simulink model "One_Stage"  (R2019b)
settings: Solver=VariableStepAuto  StartTime=0.0  StopTime=10.0  RelTol=1e-3
undefined symbols (not defined in the file): alpha, beta, hyperparameters, sigmaF, sigmaL, XFit
settings Model: Creator=licem  LastModifiedBy=licem

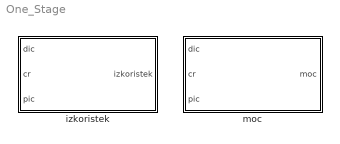
== system One_Stage ==
  izkoristek : Subsystem
  moc : Subsystem

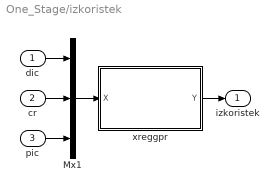
== system One_Stage/izkoristek ==
  dic : Inport
  cr : Inport  Port=2
  pic : Inport  Port=3
  Mx1 : Mux  Inputs=3
  xreggpr : Subsystem
      mask init:
      | xregmaskinitialization;
  izkoristek : Outport
  wires:
  dic/1 -> Mx1/1
  cr/1 -> Mx1/2
  pic/1 -> Mx1/3
  Mx1/1 -> xreggpr/1(X)
  xreggpr/1(Y) -> izkoristek/1

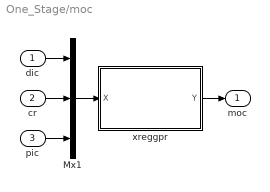
== system One_Stage/moc ==
  dic : Inport
  cr : Inport  Port=2
  pic : Inport  Port=3
  Mx1 : Mux  Inputs=3
  xreggpr : Subsystem
      mask init:
      | xregmaskinitialization;
  moc : Outport
  wires:
  dic/1 -> Mx1/1
  cr/1 -> Mx1/2
  pic/1 -> Mx1/3
  Mx1/1 -> xreggpr/1(X)
  xreggpr/1(Y) -> moc/1

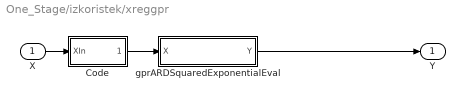
== system One_Stage/izkoristek/xreggpr ==
  X : Inport
  Code : Subsystem
  gprARDSquaredExponentialEval : Subsystem
  Y : Outport
  wires:
  X/1 -> Code/1(XIn)
  Code/1(XCoded) -> gprARDSquaredExponentialEval/1(X)
  gprARDSquaredExponentialEval/1(Y) -> Y/1

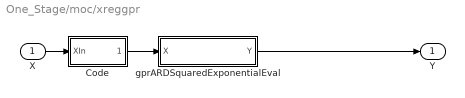
== system One_Stage/moc/xreggpr ==
  X : Inport
  Code : Subsystem
  gprARDSquaredExponentialEval : Subsystem
  Y : Outport
  wires:
  X/1 -> Code/1(XIn)
  Code/1(XCoded) -> gprARDSquaredExponentialEval/1(X)
  gprARDSquaredExponentialEval/1(Y) -> Y/1

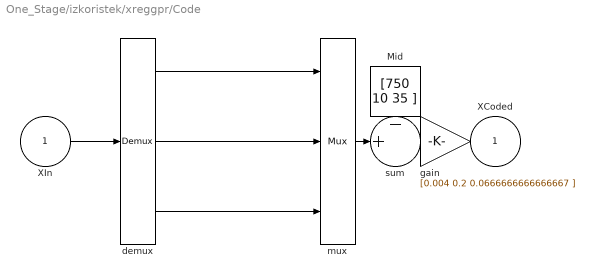
== system One_Stage/izkoristek/xreggpr/Code ==
  XIn : Inport
  Mid : Constant  Value=[750 10 35 ]
  demux : Demux  Outputs=3
  gain : Gain  Gain=[0.004 0.2 0.0666666666666667 ]  SaturateOnIntegerOverflow=on  OutDataTypeStr=Inherit: Same as input  ParamDataTypeStr=Inherit: Same as input
  mux : Mux  Inputs=3
  sum : Sum  Inputs=-+|  SaturateOnIntegerOverflow=on  InputSameDT=on  OutDataTypeStr=Inherit: Same as first input
  XCoded : Outport
  wires:
  demux/1 -> mux/1
  demux/2 -> mux/2
  demux/3 -> mux/3
  Mid/1 -> sum/1
  XIn/1 -> demux/1
  mux/1 -> sum/2
  sum/1 -> gain/1
  gain/1 -> XCoded/1

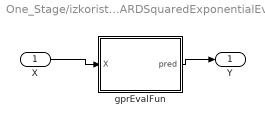
== system One_Stage/izkoristek/xreggpr/gprARDSquaredExponentialEval ==
  X : Inport
  gprEvalFun : MATLAB Function  TreatAsAtomicUnit=on
  Y : Outport
  wires:
  X/1 -> gprEvalFun/1(X)
  gprEvalFun/1(pred) -> Y/1

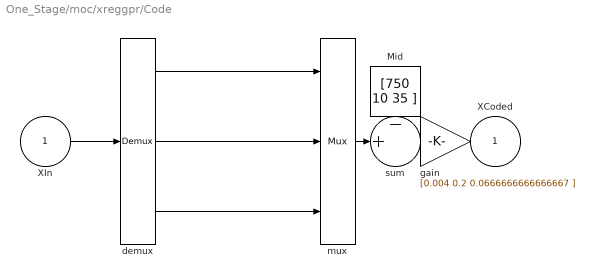
== system One_Stage/moc/xreggpr/Code ==
  XIn : Inport
  Mid : Constant  Value=[750 10 35 ]
  demux : Demux  Outputs=3
  gain : Gain  Gain=[0.004 0.2 0.0666666666666667 ]  SaturateOnIntegerOverflow=on  OutDataTypeStr=Inherit: Same as input  ParamDataTypeStr=Inherit: Same as input
  mux : Mux  Inputs=3
  sum : Sum  Inputs=-+|  SaturateOnIntegerOverflow=on  InputSameDT=on  OutDataTypeStr=Inherit: Same as first input
  XCoded : Outport
  wires:
  demux/1 -> mux/1
  demux/2 -> mux/2
  demux/3 -> mux/3
  Mid/1 -> sum/1
  XIn/1 -> demux/1
  mux/1 -> sum/2
  sum/1 -> gain/1
  gain/1 -> XCoded/1

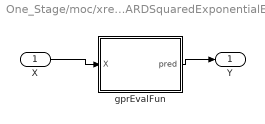
== system One_Stage/moc/xreggpr/gprARDSquaredExponentialEval ==
  X : Inport
  gprEvalFun : MATLAB Function  TreatAsAtomicUnit=on
  Y : Outport
  wires:
  X/1 -> gprEvalFun/1(X)
  gprEvalFun/1(pred) -> Y/1

== matlab function One_Stage/moc/xreggpr/gprARDSquaredExponentialEval/gprEvalFun ==
  data: X input size=nfactors; XFit parameter; alpha parameter; pred output; beta parameter; sigmaL parameter; sigmaF parameter; hyperparameters parameter
function pred = fcn(X, XFit, alpha, beta, sigmaL, sigmaF, hyperparameters)
%#codegen

% GPM evaluation for ARDSquaredExponential kernel
% X = New X value [inputs x 1]
% XFit = Fit data [inputs x #ActiveSetPoints]
% alpha = Model alpha
% beta = Model beta
% sigmaL = Length kernel parameters
% sigmaF = Signal variance
% hyperparameters = Only used by the rational quadratic kernel for its alpha hyperparameter

% Autogenerated on 27-Mar-2020 16:53:17.

% Evaluate the "ARDSquaredExponential" kernel at X
kernelAlpha = 0;
for i=1:size(XFit,1)
    ithKernel = evaluateARDSquaredExponential(X, XFit(i,:), sigmaL, sigmaF, hyperparameters);
    kernelAlpha = kernelAlpha+ithKernel*alpha(i);
end


% Create "Constant" basis
basisBeta = beta;

% Evaluate model
pred = kernelAlpha + basisBeta;


function kernelEval = evaluateARDSquaredExponential(X, XFit, sigmaL, sigmaF, hyperparameters)
% Evaluating the ARDSquaredExponential kernel for X

% Compute normalized Euclidean distances.
d = length(X);
distanceSquared = 0;
for r = 1:d
    distanceSquared = distanceSquared + (X(r)/sigmaL(r)-XFit(:,r)/sigmaL(r)).^2;
end

kernelEval = (sigmaF^2)*exp(-0.5*distanceSquared);

== matlab function One_Stage/izkoristek/xreggpr/gprARDSquaredExponentialEval/gprEvalFun ==
  data: X input size=nfactors; XFit parameter; alpha parameter; pred output; beta parameter; sigmaL parameter; sigmaF parameter; hyperparameters parameter
function pred = fcn(X, XFit, alpha, beta, sigmaL, sigmaF, hyperparameters)
%#codegen

% GPM evaluation for ARDSquaredExponential kernel
% X = New X value [inputs x 1]
% XFit = Fit data [inputs x #ActiveSetPoints]
% alpha = Model alpha
% beta = Model beta
% sigmaL = Length kernel parameters
% sigmaF = Signal variance
% hyperparameters = Only used by the rational quadratic kernel for its alpha hyperparameter

% Autogenerated on 27-Mar-2020 16:53:03.

% Evaluate the "ARDSquaredExponential" kernel at X
kernelAlpha = 0;
for i=1:size(XFit,1)
    ithKernel = evaluateARDSquaredExponential(X, XFit(i,:), sigmaL, sigmaF, hyperparameters);
    kernelAlpha = kernelAlpha+ithKernel*alpha(i);
end


% Create "Constant" basis
basisBeta = beta;

% Evaluate model
pred = kernelAlpha + basisBeta;


function kernelEval = evaluateARDSquaredExponential(X, XFit, sigmaL, sigmaF, hyperparameters)
% Evaluating the ARDSquaredExponential kernel for X

% Compute normalized Euclidean distances.
d = length(X);
distanceSquared = 0;
for r = 1:d
    distanceSquared = distanceSquared + (X(r)/sigmaL(r)-XFit(:,r)/sigmaL(r)).^2;
end

kernelEval = (sigmaF^2)*exp(-0.5*distanceSquared);
